simulink model "testemplanner_cs"  (R2020a)
settings: Solver=ode5  StartTime=0.0  StopTime=24  FixedStep=1/1000  RelTol=1e-3
PreLoadFcn:
  | mbxruntime.callbacks.PreLoadFcn(bdroot);
PostLoadFcn:
  | mbxruntime.callbacks.PostLoadFcn(bdroot);
InitFcn:
  | mbxruntime.callbacks.InitFcn(bdroot);
StartFcn:
  | mbxruntime.callbacks.StartFcn(bdroot);
StopFcn:
  | mbxruntime.callbacks.StopFcn(bdroot);
model workspace (MAT data in the model file):
  mbox_table : object (value not decoded)
  model_closed = 0
  sim_status = 0
values from neighbouring files (symbols this model uses):
  c_factor = 43.75    [emplanner_init.m]
  cf = -175016    [emplanner_init.m]
  cr = -130634    [emplanner_init.m]
  global_path_x = [0.057304 1.05668625507 2.05480936558 3.05165624935 4.04722112279 5.04150235808 6.03449985569 7.02621407764 8.01664569183 9.00579544113 9.99366409523 10.9802524329 ... (3001 elements, 3001x1)]    [global_path.mat]
  global_path_y = [8.29 8.29 8.29 8.29 8.29 8.29 8.29 8.29 8.29 8.29 8.29 8.29 ... (3001 elements, 3001x1)]    [global_path.mat]
  KD_PID_distance = 0.0    (= 0)    [emplanner_init.m]
  KD_PID_speed = 0    [emplanner_init.m]
  KI_PID_distance = 0.0    (= 0)    [emplanner_init.m]
  KI_PID_speed = 0    [emplanner_init.m]
  KP_PID_distance = 0.5    [emplanner_init.m]
  KP_PID_speed = 1.8    [emplanner_init.m]
  la = 1.265    [emplanner_init.m]
  lb = 2.947-1.265    (= 1.682)    [emplanner_init.m]
  LQR_K1 = k(:,1)'    [emplanner_init.m]
  LQR_K2 = k(:,2)'    [emplanner_init.m]
  LQR_K3 = k(:,3)'    [emplanner_init.m]
  LQR_K4 = k(:,4)'    [emplanner_init.m]
  m = 2020    [emplanner_init.m]
  rack_displacement = [-39.14 , -37.2 , -35.29 , -33.43 , -31.6 , -29.81 , -28.06 , -26.34 , -24.66 ,      -23.01 , -21.38 , -19.79 , -18.23 , -16.69 , -15.18 , -13.7 , -12.23 , -10.8 , -9.38 , -7.98 ,     -6.61 , -5.25 , -3.91 , -2.59 , -1.29 , 0 , 1.27 , 2.54 , 3.78 , 5.02 , 6.24 , 7.46 , 8.66 ,      9.86 , 11.05 , 12.24 , 13.41 , 14.59 , 15.76 , 16.92 , 18.09 , 19.25 , 20.42 , 21.59 , 22.76 ,      23.93 , 25.11 , 26 ...(+26 chars)    [emplanner_init.m]
  right_wheel_ground = [-70 ,-67.2 , -64.4 , -61.6 , -58.8 , -56 , -53.2 , -50.4 , -47.6 , -44.8 , -42 ,      -39.2 , -36.4 , -33.6 , -30.8 , -28 , -25.2 , -22.4 , -19.6 , -16.8 , -14 , -11.2 , -8.4 , -5.6 ,      -2.8 , 0 , 2.8 , 5.6 , 8.4 , 11.2 , 14 , 16.8 , 19.6 , 22.4 , 25.2 , 28 , 30.8 , 33.6 , 36.4 ,      39.2 , 42 , 44.8 , 47.6 , 50.4 , 53.2 , 56 , 58.8 , 61.6 , 64.4 , 67.2 , 70 ]    [emplanner_init.m]
  vx_break_point = zeros(1,5000)    [emplanner_init.m]
undefined symbols (not defined in the file or in its folder): aubr, DiscIntNeverNeededParam, tablebr, vubr
libraries: PreScanSimulinkLibrary x9, Solver_SF x1, simulink_extras x1
(part 5 of 9)

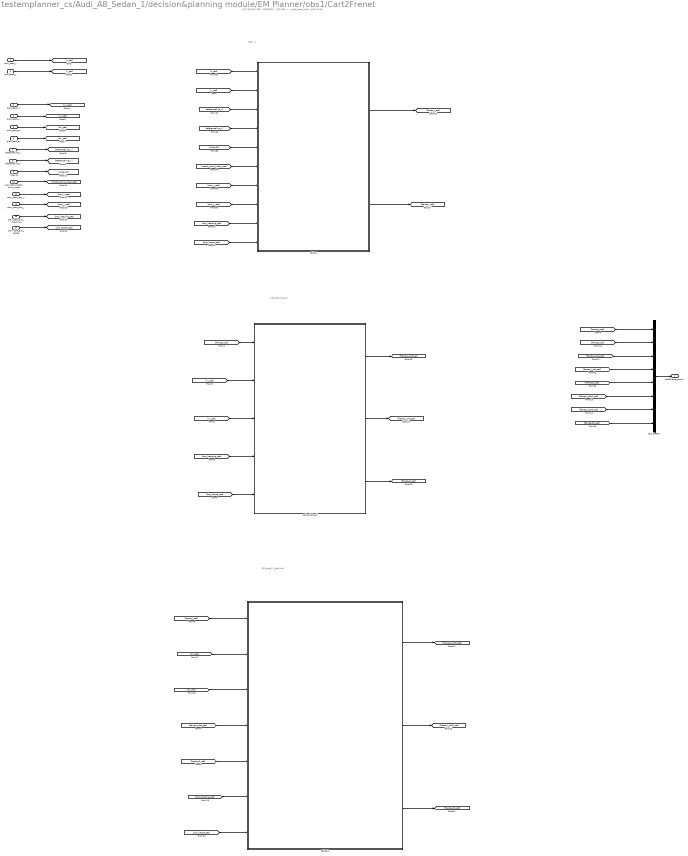
== system testemplanner_cs/Audi_A8_Sedan_1/decision&planning module/EM Planner/obs1/Cart2Frenet ==
  note: 计算s_dot_2,l_dot2,ddl
  note: 计算s_dot,l_dot,dl
  note: 计算S，L
  note: 分成三部分进行计算，方便后续拆分，分别计算S，L，s_dot,l_dot,s_dot2,l_dot2,dl和ddl
  plan_start_x : Inport
  plan_start_y : Inport  Port=2
  plan_start_vx : Inport  Port=3
  plan_start_vy : Inport  Port=4
  plan_start_ax : Inport  Port=5
  plan_start_ay : Inport  Port=6
  referenceline_x : Inport  Port=7
  referenceline_y : Inport  Port=8
  index2s : Inport  Port=9
  plan_start_match_point_index : Inport  Port=10
  plan_start_proj_x : Inport  Port=11
  plan_start_proj_y : Inport  Port=12
  plan_start_proj_heading : Inport  Port=13
  plan_start_proj_kappa : Inport  Port=14
  Bus Creator : BusCreator  Inputs=8
  CalcSL : MATLAB Function  TreatAsAtomicUnit=on
  CalcSL2 : MATLAB Function  TreatAsAtomicUnit=on
  Calcs_l_dot_dl : MATLAB Function  TreatAsAtomicUnit=on
  Cart2Frenet_result : Outport
  wires:
  Bus Creator/1 -> Cart2Frenet_result/1
  [frenet_ddl_set] -> Bus Creator/8
  [frenet_l_dot2_set] -> Bus Creator/7
  [frenet_s_dot2_set] -> Bus Creator/6
  [frenet_dl_set] -> Bus Creator/5
  [frenet_l_dot_set] -> Bus Creator/4
  [frenet_s_dot_set] -> Bus Creator/3
  [frenet_l_set] -> Bus Creator/2
  [frenet_s_set] -> Bus Creator/1
  CalcSL2/1(s_dot2_set) -> [frenet_s_dot2_set]
  CalcSL2/2(l_dot2_set) -> [frenet_l_dot2_set]
  CalcSL2/3(ddl_set) -> [frenet_ddl_set]
  [frenet_s_dot_set] -> CalcSL2/4(s_dot_set)
  [frenet_l_set] -> CalcSL2/1(frenet_l_set)
  [frenet_dl_set] -> CalcSL2/5(dl_set)
  [ay_set] -> CalcSL2/3(ay_set)
  [ax_set] -> CalcSL2/2(ax_set)
  Calcs_l_dot_dl/3(dl_set) -> [frenet_dl_set]
  Calcs_l_dot_dl/2(l_dot_set) -> [frenet_l_dot_set]
  Calcs_l_dot_dl/1(s_dot_set) -> [frenet_s_dot_set]
  [vy_set] -> Calcs_l_dot_dl/3(vy_set)
  [frenet_l_set] -> Calcs_l_dot_dl/1(frenet_l_set)
  CalcSL/2(frenet_l_set) -> [frenet_l_set]
  [proj_kappa_set] -> CalcSL2/7(plan_start_proj_kappa)
  [proj_heading_set] -> CalcSL2/6(plan_start_proj_heading)
  [vx_set] -> Calcs_l_dot_dl/2(vx_set)
  [proj_heading_set] -> Calcs_l_dot_dl/4(plan_start_proj_heading)
  [proj_kappa_set] -> Calcs_l_dot_dl/5(plan_start_proj_kappa)
  [proj_kappa_set] -> CalcSL/10(plan_start_proj_kappa)
  [proj_heading_set] -> CalcSL/9(plan_start_proj_heading)
  [proj_y_set] -> CalcSL/8(plan_start_proj_y)
  [proj_x_set] -> CalcSL/7(plan_start_proj_x)
  [match_point_index_set] -> CalcSL/6(plan_start_match_point_index)
  [index2s] -> CalcSL/5(index2s)
  [referenceline_y] -> CalcSL/4(referenceline_y)
  [referenceline_x] -> CalcSL/3(referenceline_x)
  [y_set] -> CalcSL/2(y_set)
  [x_set] -> CalcSL/1(x_set)
  plan_start_proj_kappa/1 -> [proj_kappa_set]
  plan_start_proj_heading/1 -> [proj_heading_set]
  plan_start_proj_y/1 -> [proj_y_set]
  plan_start_proj_x/1 -> [proj_x_set]
  plan_start_match_point_index/1 -> [match_point_index_set]
  index2s/1 -> [index2s]
  referenceline_y/1 -> [referenceline_y]
  referenceline_x/1 -> [referenceline_x]
  plan_start_ay/1 -> [ay_set]
  plan_start_ax/1 -> [ax_set]
  plan_start_vy/1 -> [vy_set]
  plan_start_vx/1 -> [vx_set]
  plan_start_y/1 -> [y_set]
  plan_start_x/1 -> [x_set]
  CalcSL/1(frenet_s_set) -> [frenet_s_set]

== system testemplanner_cs/Audi_A8_Sedan_1/decision&planning module/EM_planner1/obs/Cart2Frenet ==
  note: 计算s_dot_2,l_dot2,ddl
  note: 计算s_dot,l_dot,dl
  note: 计算S，L
  note: 分成三部分进行计算，方便后续拆分，分别计算S，L，s_dot,l_dot,s_dot2,l_dot2,dl和ddl
  plan_start_x : Inport
  plan_start_y : Inport  Port=2
  plan_start_vx : Inport  Port=3
  plan_start_vy : Inport  Port=4
  plan_start_ax : Inport  Port=5
  plan_start_ay : Inport  Port=6
  referenceline_x : Inport  Port=7
  referenceline_y : Inport  Port=8
  index2s : Inport  Port=9
  plan_start_match_point_index : Inport  Port=10
  plan_start_proj_x : Inport  Port=11
  plan_start_proj_y : Inport  Port=12
  plan_start_proj_heading : Inport  Port=13
  plan_start_proj_kappa : Inport  Port=14
  Bus Creator : BusCreator  Inputs=8
  CalcSL : MATLAB Function  TreatAsAtomicUnit=on
  CalcSL2 : MATLAB Function  TreatAsAtomicUnit=on
  Calcs_l_dot_dl : MATLAB Function  TreatAsAtomicUnit=on
  Cart2Frenet_result : Outport
  wires:
  Bus Creator/1 -> Cart2Frenet_result/1
  [frenet_ddl_set] -> Bus Creator/8
  [frenet_l_dot2_set] -> Bus Creator/7
  [frenet_s_dot2_set] -> Bus Creator/6
  [frenet_dl_set] -> Bus Creator/5
  [frenet_l_dot_set] -> Bus Creator/4
  [frenet_s_dot_set] -> Bus Creator/3
  [frenet_l_set] -> Bus Creator/2
  [frenet_s_set] -> Bus Creator/1
  CalcSL2/1(s_dot2_set) -> [frenet_s_dot2_set]
  CalcSL2/2(l_dot2_set) -> [frenet_l_dot2_set]
  CalcSL2/3(ddl_set) -> [frenet_ddl_set]
  [frenet_s_dot_set] -> CalcSL2/4(s_dot_set)
  [frenet_l_set] -> CalcSL2/1(frenet_l_set)
  [frenet_dl_set] -> CalcSL2/5(dl_set)
  [ay_set] -> CalcSL2/3(ay_set)
  [ax_set] -> CalcSL2/2(ax_set)
  Calcs_l_dot_dl/3(dl_set) -> [frenet_dl_set]
  Calcs_l_dot_dl/2(l_dot_set) -> [frenet_l_dot_set]
  Calcs_l_dot_dl/1(s_dot_set) -> [frenet_s_dot_set]
  [vy_set] -> Calcs_l_dot_dl/3(vy_set)
  [frenet_l_set] -> Calcs_l_dot_dl/1(frenet_l_set)
  CalcSL/2(frenet_l_set) -> [frenet_l_set]
  [proj_kappa_set] -> CalcSL2/7(plan_start_proj_kappa)
  [proj_heading_set] -> CalcSL2/6(plan_start_proj_heading)
  [vx_set] -> Calcs_l_dot_dl/2(vx_set)
  [proj_heading_set] -> Calcs_l_dot_dl/4(plan_start_proj_heading)
  [proj_kappa_set] -> Calcs_l_dot_dl/5(plan_start_proj_kappa)
  [proj_kappa_set] -> CalcSL/10(plan_start_proj_kappa)
  [proj_heading_set] -> CalcSL/9(plan_start_proj_heading)
  [proj_y_set] -> CalcSL/8(plan_start_proj_y)
  [proj_x_set] -> CalcSL/7(plan_start_proj_x)
  [match_point_index_set] -> CalcSL/6(plan_start_match_point_index)
  [index2s] -> CalcSL/5(index2s)
  [referenceline_y] -> CalcSL/4(referenceline_y)
  [referenceline_x] -> CalcSL/3(referenceline_x)
  [y_set] -> CalcSL/2(y_set)
  [x_set] -> CalcSL/1(x_set)
  plan_start_proj_kappa/1 -> [proj_kappa_set]
  plan_start_proj_heading/1 -> [proj_heading_set]
  plan_start_proj_y/1 -> [proj_y_set]
  plan_start_proj_x/1 -> [proj_x_set]
  plan_start_match_point_index/1 -> [match_point_index_set]
  index2s/1 -> [index2s]
  referenceline_y/1 -> [referenceline_y]
  referenceline_x/1 -> [referenceline_x]
  plan_start_ay/1 -> [ay_set]
  plan_start_ax/1 -> [ax_set]
  plan_start_vy/1 -> [vy_set]
  plan_start_vx/1 -> [vx_set]
  plan_start_y/1 -> [y_set]
  plan_start_x/1 -> [x_set]
  CalcSL/1(frenet_s_set) -> [frenet_s_set]

== system testemplanner_cs/Audi_A8_Sedan_1/Trajectories/Traj2State1/Traj2State2/Traj2MuxState_Ext/demux ==
  traj : Inport
  Demux : Demux  Outputs=18
  x : Outport
  y : Outport  Port=2
  z : Outport  Port=3
  velx : Outport  Port=4
  vely : Outport  Port=5
  velz : Outport  Port=6
  R : Outport  Port=7
  P : Outport  Port=8
  Y : Outport  Port=9
  velR : Outport  Port=10
  velP : Outport  Port=11
  velY : Outport  Port=12
  accx : Outport  Port=13
  accy : Outport  Port=14
  accz : Outport  Port=15
  accR : Outport  Port=16
  accP : Outport  Port=17
  accY : Outport  Port=18
  wires:
  Demux/18 -> accY/1
  Demux/17 -> accP/1
  Demux/16 -> accR/1
  Demux/15 -> accz/1
  Demux/14 -> accy/1
  Demux/13 -> accx/1
  Demux/12 -> velY/1
  Demux/11 -> velP/1
  Demux/10 -> velR/1
  Demux/9 -> velz/1
  Demux/8 -> vely/1
  Demux/7 -> velx/1
  Demux/6 -> Y/1
  Demux/5 -> P/1
  traj/1 -> Demux/1
  Demux/4 -> R/1
  Demux/3 -> z/1
  Demux/2 -> y/1
  Demux/1 -> x/1

== matlab function testemplanner_cs/Audi_A8_Sedan_1/decision&planning module/EM_planner1/calc speed planning start condition ==
  data: plan_start_vx input; plan_start_s_dot output; plan_start_vy input; plan_start_ax input; plan_start_ay input; plan_start_heading input; plan_start_s_dot2 output
function [plan_start_s_dot,plan_start_s_dot2] = fcn(plan_start_vx,plan_start_vy,plan_start_ax,plan_start_ay,plan_start_heading)
% 该函数计算速度规划的初始条件
tor = [cos(plan_start_heading);sin(plan_start_heading)];
v_t = tor'*[plan_start_vx;plan_start_vy];
a_t = tor'*[plan_start_ax;plan_start_ay];
plan_start_s_dot = v_t;
plan_start_s_dot2 = a_t;

== matlab function testemplanner_cs/Audi_A8_Sedan_1/decision&planning module/EM Planner/Cartesian2Frenet1/MATLAB Function2 ==
  data: ax_set input; s_dot2_set output; ay_set input; proj_heading_set input; proj_kappa_set input; l_set input; s_dot_set input; dl_set input; l_dot2_set output; ddl_set output
function [s_dot2_set,l_dot2_set,ddl_set] = fcn(ax_set,ay_set,proj_heading_set,proj_kappa_set,l_set,s_dot_set,dl_set)
%由于不知道有多少个点需要做坐标转换，设一个最大值做缓冲
n = 128;
% 输出初始化
s_dot2_set = ones(n,1)*nan;
l_dot2_set = ones(n,1)*nan;
ddl_set = ones(n,1)*nan;

for i = 1:length(l_set)
    if isnan(l_set(i))
       break;
    end
    a_h = [ax_set(i);ay_set(i)];
    n_r = [-sin(proj_heading_set(i));cos(proj_heading_set(i))];
    t_r = [cos(proj_heading_set(i));sin(proj_heading_set(i))];
    %近似认为dkr/ds 为0 简化计算
    l_dot2_set(i) = a_h'*n_r - proj_kappa_set(i) * (1 - proj_kappa_set(i) * l_set(i)) * s_dot_set(i)^2;
    s_dot2_set(i) = (1/(1 - proj_kappa_set(i) * l_set(i)))* (a_h' * t_r + 2 * proj_kappa_set(i) * dl_set(i) * s_dot_set(i)^2);
    % 要考虑加速度为0的情况
    if (s_dot2_set(i) < 1e-6)
        ddl_set(i) = 0;
    else
        ddl_set(i) = (l_dot2_set(i) - dl_set(i)*s_dot2_set(i))/(s_dot_set(i)^2);
    end
end

== matlab function testemplanner_cs/Audi_A8_Sedan_1/decision&planning module/EM_planner1/general fast algorithm to find projection point info3 ==
  data: x_set input; match_point_index_set output; y_set input; path_x input; path_y input; proj_x_set output; proj_y_set output; proj_heading_set output; proj_kappa_set output; path_heading input; path_kappa input
function [match_point_index_set,proj_x_set,proj_y_set,proj_heading_set,proj_kappa_set] = fcn(x_set,y_set,path_x,path_y,path_heading,path_kappa)
%该函数是一个通用函数，找到x_set,y_set在path_x,path_y的匹配点的编号，以及投影点在直角坐标系下的(x,y,theta,kappa)
%最多可以处理128个点

match_point_index_set = ones(128,1)*nan;
proj_x_set = ones(128,1)*nan;
proj_y_set = ones(128,1)*nan;
proj_heading_set = ones(128,1)*nan;
proj_kappa_set = ones(128,1)*nan;

persistent is_first_run;
persistent init_search_index_set;
persistent pre_frenet_path_x;
persistent pre_frenet_path_y;
persistent pre_frenet_path_heading;
persistent pre_frenet_path_kappa;
if isempty(is_first_run)
    is_first_run = 0; 
    init_search_index_set = ones(128,1)*nan;
    start_index = 1;
    pre_frenet_path_x = path_x;
    pre_frenet_path_y = path_y;
    pre_frenet_path_heading = path_heading;
    pre_frenet_path_kappa = path_kappa;
    for i = 1:length(x_set)
        if isnan(x_set(i))
            break;
        else
            increase_count = 0;
            min_distance = 1e10;
            for j = start_index:length(path_x)
                distance = (x_set(i)-path_x(j))^2 + (y_set(i)-path_y(j))^2;
                if (min_distance > distance)
                    min_distance = distance;
                    match_point_index_set(i)=j;
                    increase_count = 0;
                else
                    increase_count = increase_count + 1;
                end
                if increase_count > 50
                    break;
                end
            end
            match_point_index = match_point_index_set(i);
            vector_match_point = [path_x(match_point_index);path_y(match_point_index)];
            vector_match_point_direction = [cos(path_heading(match_point_index));sin(path_heading(match_point_index))];
            vector_host_point = [x_set(i);y_set(i)];
            vector_d = vector_host_point - vector_match_point;
            vector_err = (vector_d'* vector_match_point_direction) * vector_match_point_direction;
            vector_proj = vector_err + vector_match_point;
            proj_x_set(i) = vector_proj(1);
            proj_y_set(i) = vector_proj(2);
            proj_heading_set(i) = path_heading(match_point_index) + path_kappa(match_point_index) * (vector_d'* vector_match_point_direction);
            proj_kappa_set(i) = path_kappa(match_point_index);            
        end
    end 
    init_search_index_set=match_point_index_set;
else
    min_distance = inf;
    for i = 1:length(x_set)
        increase_count = 0;
        count_limit=5;
        if isnan(init_search_index_set(i))
            start_index = 1;
            count_limit=50;
       
        
        else
            
            start_index = init_search_index_set(i);
          
         end  
            
            vector_m_init = [pre_frenet_path_x(start_index);pre_frenet_path_y(start_index)];
            vector_direction_init = [cos(pre_frenet_path_heading(start_index));sin(pre_frenet_path_heading(start_index))];
            ds = vector_m_init'*vector_direction_init;
            if ds > 0.001            
                for j = start_index:length(pre_frenet_path_x )
                    distance = (x_set(i)-pre_frenet_path_x (j))^2 + (y_set(i)-pre_frenet_path_y(j))^2;
                    if (min_distance > distance)
                        min_distance = distance;
                        init_search_index_set(i)=j;
                        increase_count = 0;
                    else
                        increase_count = increase_count + 1;
                    end
                    if increase_count > count_limit
                        break;
                    end
                end
            elseif ds < -0.001
                for j = start_index:-1:1
                    distance = (x_set(i)-pre_frenet_path_x (j))^2 + (y_set(i)-pre_frenet_path_y(j))^2;
                    if (min_distance > distance)
                        min_distance = distance;
                        init_search_index_set(i)=j;
                        increase_count = 0;
                    else
                        increase_count = increase_count + 1;
                    end
                    if increase_count >  count_limit
                        break;
                    end
                end
              match_point_index_set(i)=start_index;  
            end
            
           match_point_index= match_point_index_set(i);
            vector_match_point = [pre_frenet_path_x(match_point_index);pre_frenet_path_y(match_point_index)];
            vector_match_point_direction = [cos(pre_frenet_path_heading(match_point_index));sin(pre_frenet_path_heading(match_point_index))];
            vector_host_point = [x_set(i);y_set(i)];
            vector_d = vector_host_point - vector_match_point;
            vector_err = (vector_d'* vector_match_point_direction) * vector_match_point_direction;
            vector_proj = vector_err + vector_match_point;
            proj_x_set(i) = vector_proj(1);
            proj_y_set(i) = vector_proj(2);
            proj_heading_set(i) = pre_frenet_path_heading(match_point_index) + pre_frenet_path_kappa(match_point_index) * (vector_d'* vector_match_point_direction);
            proj_kappa_set(i) = pre_frenet_path_kappa(match_point_index);            
        end
    end    
    init_search_index_set = match_point_index_set;
    pre_frenet_path_x = path_x;
    pre_frenet_path_y = path_y;
    pre_frenet_path_heading = path_heading;
    pre_frenet_path_kappa = path_kappa;
end

== matlab function testemplanner_cs/Audi_A8_Sedan_1/decision&planning module/EM_planner1/increase st point count ==
  data: s_init input; s output; s_dot_init input; s_dot2_init input; relative_time_init input; s_dot output; s_dot2 output; relative_time output
function [s,s_dot,s_dot2,relative_time] = fcn(s_init,s_dot_init,s_dot2_init,relative_time_init)
%该函数将增密s s_dot s_dot2
% 为什么需要增密，因为控制的执行频率是规划的10倍，轨迹点如果不够密，必然会导致规划效果不好
% 但是若在速度二次规划中点取的太多，会导致二次规划的矩阵规模太大计算太慢
% 所以方法是在二次规划中选取少量的点优化完毕后，在用此函数增密
T = relative_time_init(end);
n = 401;
dt = T/(n-1);
s = zeros(n,1);
s_dot = zeros(n,1);
s_dot2 = zeros(n,1);
relative_time = zeros(n,1);
for i = 1:n
    current_t = (i-1)*dt;
    for j = 1:length(relative_time_init)-1
        if relative_time_init(j) <= current_t && relative_time_init(j+1) > current_t
            break;
        end
    end
    x = current_t - relative_time_init(j);
    s(i) = s_init(j) + s_dot_init(j)*x + (1/3)*s_dot2_init(j)*x^2 + (1/6)*s_dot2_init(j+1)*x^2; 
    s_dot(i) = s_dot_init(j) + 0.5*s_dot2_init(j)*x + 0.5*s_dot2_init(j+1)*x;
    s_dot2(i) = s_dot2_init(j) + (s_dot2_init(j+1) - s_dot2_init(j))*x/(relative_time_init(j+1) - relative_time_init(j));
    relative_time(i) = current_t;
end

== matlab function testemplanner_cs/Audi_A8_Sedan_1/decision&planning module/EM_planner1/obs/Cart2Frenet/CalcSL ==
  data: x_set input; y_set input; referenceline_x input; referenceline_y input; index2s input; plan_start_match_point_index input; plan_start_proj_x input; plan_start_proj_y input; plan_start_proj_heading input; plan_start_proj_kappa input; frenet_s_set output; frenet_l_set output
function [frenet_s_set,frenet_l_set] =fcn(x_set,y_set,referenceline_x,referenceline_y,index2s,plan_start_match_point_index,plan_start_proj_x,plan_start_proj_y,plan_start_proj_heading,plan_start_proj_kappa)
%作用：这是一个通用函数，计算输入的笛卡尔坐标点x,y在自然坐标（frenet）坐标系中的s和l
%输入:要计算的点集的x,y坐标，航向，曲率。他的投影点的x,y坐标，index2s数据，以及参考线数据
%输出：自然坐标系下的s和l
%首先对s和l做一个缓冲
frenet_s_set=ones(128,1)*nan;
frenet_l_set=ones(128,1)*nan;
%开始计算
for i=1:length(x_set)
if isnan(x_set(i))  %遇到空的跳出
    break;
end
%调用相关函数进行s的计算
frenet_s_set(i)=CalcSfromIndex(referenceline_x,referenceline_y,plan_start_proj_x(i),plan_start_proj_y(i),plan_start_match_point_index(i),index2s);

%进行l的计算
%先求自然坐标系的切向量和法向量
%切向量,没用到
%tor=[cos(plan_start_proj_heading(i));sin(plan_start_proj_heading(i))];
%法向量
nor=[-sin(plan_start_proj_heading(i));cos(plan_start_proj_heading(i))];
frenet_l_set(i)=[x_set(i)-plan_start_proj_x(i);y_set(i)-plan_start_proj_y(i)]'*nor;
end

end
function s=CalcSfromIndex(ref_path_x,ref_path_y,match_point_x,match_point_y,match_point_index,index2s)   %使用一个函数来计算index所对应的S值
%%首先判断原点是在匹配点前还是匹配点后，通过向量的内积来进行判断
s_temp =  index2s(match_point_index);
vector1=[match_point_x-ref_path_x(match_point_index);match_point_y-ref_path_y(match_point_index)];
%考虑匹配点在路径终点的情况，不在终点就是匹配点和下一个点作为方向向量，如果是终点则使用匹配点和上一个点作为方向向量
if match_point_index<length(ref_path_x)
    vector2=[ref_path_x(match_point_index+1)-ref_path_x(match_point_index);ref_path_y(match_point_index+1)-ref_path_y(match_point_index)];
else
     vector2=[ref_path_x(match_point_index)-ref_path_x(match_point_index-1);ref_path_y(match_point_index)-ref_path_y(match_point_index-1)];
end
result=vector1'*vector2;    
if result >0 %原点在匹配点后，加上这个距离
    s=s_temp+sqrt(vector1'*vector1);
else        %原点在匹配点前，减去这个距离
    s=s_temp-sqrt(vector1'*vector1);
end
end

== matlab function testemplanner_cs/Audi_A8_Sedan_1/decision&planning module/EM_planner1/obs/Cart2Frenet/CalcSL2 ==
  data: frenet_l_set input; ax_set input; ay_set input; s_dot_set input; dl_set input; plan_start_proj_heading input; plan_start_proj_kappa input; s_dot2_set output; l_dot2_set output; ddl_set output
function [ s_dot2_set, l_dot2_set,ddl_set]=fcn(frenet_l_set,ax_set,ay_set,s_dot_set,dl_set,plan_start_proj_heading,plan_start_proj_kappa)
%作用：通过之前计算得到的l，s_dot、dl值以及已知的ax，ay值，计算s_dot2,l_dot2,以及ddl
 %首先做一个缓冲
 n=128;
 s_dot2_set=ones(n,1)*nan;
 l_dot2_set=ones(n,1)*nan;
 ddl_set=ones(n,1)*nan;

 for i=1:length(frenet_l_set)
     if isnan(frenet_l_set(i))
         break;
     end
    %先求自然坐标系的切向量和法向量
%切向量
tor=[cos(plan_start_proj_heading(i));sin(plan_start_proj_heading(i))];
%法向量
nor=[-sin(plan_start_proj_heading(i));cos(plan_start_proj_heading(i))];

ah=[ax_set(i);ay_set(i)];
l_dot2_set(i)=ah'*nor- plan_start_proj_kappa(i) * (1 - plan_start_proj_kappa(i) * frenet_l_set(i)) * s_dot_set(i)^2;
s_dot2_set(i)=(1/(1 - plan_start_proj_kappa(i) * frenet_l_set(i)))* (ah' * tor + 2 * plan_start_proj_kappa(i) * dl_set(i) * s_dot_set(i)^2);

if abs(s_dot2_set(i))<1e-6
    ddl_set(i)=0;
else
    ddl_set(i)=(l_dot2_set(i) - dl_set(i)*s_dot2_set(i))/(s_dot_set(i)^2);
 end
end

== matlab function testemplanner_cs/Audi_A8_Sedan_1/decision&planning module/EM_planner1/obs/Cart2Frenet/Calcs_l_dot_dl ==
  data: frenet_l_set input; vx_set input; vy_set input; plan_start_proj_heading input; plan_start_proj_kappa input; s_dot_set output; l_dot_set output; dl_set output
function [ s_dot_set, l_dot_set,dl_set]=fcn(frenet_l_set,vx_set,vy_set,plan_start_proj_heading,plan_start_proj_kappa)
%作用：通过之前计算得到的s和l值以及计算的速度值，计算s_dot,l_dot,以及dl
 %首先做一个缓冲
 n=128;
 s_dot_set=ones(n,1)*nan;
 l_dot_set=ones(n,1)*nan;
 dl_set=ones(n,1)*nan;

 for i=1:length(frenet_l_set)
     if isnan(frenet_l_set(i))
         break;
     end
    %先求自然坐标系的切向量和法向量
%切向量
tor=[cos(plan_start_proj_heading(i));sin(plan_start_proj_heading(i))];
%法向量
nor=[-sin(plan_start_proj_heading(i));cos(plan_start_proj_heading(i))];

vh=[vx_set(i);vy_set(i)];
l_dot_set(i)=vh'*nor;
s_dot_set(i)=vh'*tor/(1-plan_start_proj_kappa(i)*frenet_l_set(i));

if abs(s_dot_set(i))<1e-6
    dl_set(i)=0;
else
    dl_set(i)=l_dot_set(i)/s_dot_set(i);
 end
end

== matlab function testemplanner_cs/Audi_A8_Sedan_1/decision&planning module/EM_planner1/obs/MATLAB Function2 ==
  data: x_set input; match_point_index_set output; y_set input; frenet_path_x input; frenet_path_y input; frenet_path_heading input; frenet_path_kappa input; proj_x_set output; proj_y_set output; proj_heading_set output; proj_kappa_set output
function [match_point_index_set,proj_x_set, proj_y_set,proj_heading_set,proj_kappa_set] = ...
    fcn(x_set,y_set,frenet_path_x,frenet_path_y,frenet_path_heading,frenet_path_kappa)
%该函数将批量计算x_set，y_set中的xy，在frenet_path下的投影的信息
%输入 x_set,y_set，待投影的点的集合
%x_set,y_set,frenet_path_x,frenet_path_y,frenet_path_heading,frenet_path_kappa
%曲线在直角坐标系下的x，y，heading，kappa
%输出：match_point_index_set 匹配点在frenet_path下的编号的集合(即从全局路径第一个点开始数，第几个点是匹配点)
%     proj_x y heading kappa 投影的x,y,heading,kappa的集合

% 由于事先不知道x_set中到底有多少个点需要投影，因此事先声明一个最大的数量的点作为缓冲
n = 128;
% 并且由于不知道投影点的个数，所以也不知道输出的个数，因此输出也要做缓冲，用nan表示不存在的点
% 输出最多输出128个
% 输出初始化
match_point_index_set = ones(n,1) * nan;
proj_x_set = ones(n,1) * nan;
proj_y_set = ones(n,1) * nan;
proj_heading_set = ones(n,1) * nan;
proj_kappa_set = ones(n,1) * nan;

%找匹配点，需要利用上一个周期的结果作为下一个周期遍历的起点，因此需要声明两个全局变量
persistent is_first_run;
persistent pre_match_point_index_set;
persistent pre_frenet_path_x;
persistent pre_frenet_path_y;
persistent pre_frenet_path_heading;
persistent pre_frenet_path_kappa;
%算法主函数入口

if isempty(is_first_run)
    %该if分支表示函数首次运行
    is_first_run = 0;
    pre_frenet_path_x = frenet_path_x;
    pre_frenet_path_y = frenet_path_y;
    pre_frenet_path_heading = frenet_path_heading;
    pre_frenet_path_kappa = frenet_path_kappa;
    %要记录首次运行计算的匹配点的结果供下个周期运行，先初始化
    pre_match_point_index_set = ones(n,1) * nan;
    %对x_set,y_set的点做遍历，找到他们的匹配点
    for i = 1 : length(x_set)
        if isnan(x_set(i))
            break;
        end
        %首次运行时，没有任何提示，只能从frenet path的第一个点开始找
        start_search_index = 1;
        % 声明increase_count，用于表示在遍历时distance连续增加的个数
        increase_count = 0;
        % 开始遍历
        min_distance = inf;
        for j = start_search_index : length(frenet_path_x)
            distance = (x_set(i) - frenet_path_x(j))^2 + (y_set(i) - frenet_path_y(j))^2;
            if distance < min_distance
                min_distance = distance;
                match_point_index_set(i) = j;
                increase_count = 0;
            else
                increase_count = increase_count + 1;
            end
            %如果distance连续增加50次就不要再遍历了，节省时间
            if increase_count > 50
                break;
            end
        end
        
        %如何通过匹配点计算投影点，请参见《自动驾驶控制算法第七讲》
        %或《自动驾驶决策规划算法》第一章第三节
        
        %取出匹配点的编号
        match_point_index = match_point_index_set(i);
        %取出匹配点的信息
        match_point_x = frenet_path_x(match_point_index);
        match_point_y = frenet_path_y(match_point_index);
        match_point_heading = frenet_path_heading(match_point_index);
        match_point_kappa = frenet_path_kappa(match_point_index);
        %计算匹配点的方向向量与法向量
        vector_match_point = [match_point_x;match_point_y];
        vector_match_point_direction = [cos(match_point_heading);sin(match_point_heading)];
        %声明待投影点的位矢
        vector_r = [x_set(i);y_set(i)];
        
       %通过匹配点计算投影点
       vector_d = vector_r - vector_match_point;
       ds = vector_d' * vector_match_point_direction;
       vector_proj_point = vector_match_point + ds * vector_match_point_direction;
       proj_heading = match_point_heading + match_point_kappa * ds;
       proj_kappa = match_point_kappa;
       %计算结果输出
       proj_x_set(i) = vector_proj_point(1);
       proj_y_set(i) = vector_proj_point(2);
       proj_heading_set(i) = proj_heading;
       proj_kappa_set(i) = proj_kappa;
    end
    %匹配点的计算结果保存，供下一个周期使用
    pre_match_point_index_set = match_point_index_set;
else
    %此if分支表示不是首次运行
    
    %对每个x_set上的点做处理
    for i = 1 : length(x_set)
        %不是首次运行，对于点x_set(i),y_set(i)来说,start_search_index =
        %pre_match_point_index_set(i)
        start_search_index = pre_match_point_index_set(i);%上个周期匹配点的编号作为本周期搜索的起点
        % 声明increase_count，用于表示在遍历时distance连续增加的个数
        %%%%%%%%%
        %对于障碍物检测而言，当感知第一次检测到障碍物时，算法并不是首次运行，此时 
        %pre_match_point_index_set的值是nan，如果还用上一时刻的结果作为本周期搜索的起点
        %必然会出问题，所以要修改
        % 声明increase_count_limit
        increase_count_limit = 5;
        if isnan(start_search_index)
            %没有上个周期的结果，那就不能只检查5次了
            increase_count_limit = 50;
            %搜索起点也要设为1
            start_search_index = 1;
        end
        increase_count = 0;
        % 开始遍历
        %这里多一个步骤，判断遍历的方向
        %计算上个周期匹配点的位矢
        vector_pre_match_point = [pre_frenet_path_x(start_search_index);pre_frenet_path_y(start_search_index)];
        vector_pre_match_point_direction = ...
            [cos(pre_frenet_path_heading(start_search_index));sin(pre_frenet_path_heading(start_search_index))];
        %判断遍历的方向
        flag = ([x_set(i);y_set(i)] - vector_pre_match_point)' * vector_pre_match_point_direction;
        min_distance = inf;
        if flag > 0.001
            for j = start_search_index : length(frenet_path_x)
                distance = (x_set(i) - frenet_path_x(j))^2 + (y_set(i) - frenet_path_y(j))^2;
                if distance < min_distance
                    min_distance = distance;
                    match_point_index_set(i) = j;
                    increase_count = 0;
                else
                    increase_count = increase_count + 1;
                end
                %如果distance连续增加increase_count_limit次就不要再遍历了，节省时间
                if increase_count > increase_count_limit
                    break;
                end
            end
        elseif flag < - 0.001
            for j = start_search_index : -1 : 1
                distance = (x_set(i) - frenet_path_x(j))^2 + (y_set(i) - frenet_path_y(j))^2;
                if distance < min_distance
                    min_distance = distance;
                    match_point_index_set(i) = j;
                    increase_count = 0;
                else
                    increase_count = increase_count + 1;
                end
                %如果distance连续增加increase_count_limit次就不要再遍历了，节省时间
                if increase_count > increase_count_limit
                    break;
                end
            end
        else
            match_point_index_set(i) = start_search_index;
        end
        
        %如何通过匹配点计算投影点，请参见《自动驾驶控制算法第七讲》
        %或《自动驾驶决策规划算法》第一章第三节
        
        %取出匹配点的编号
        match_point_index = match_point_index_set(i);
        %取出匹配点的信息
        match_point_x = frenet_path_x(match_point_index);
        match_point_y = frenet_path_y(match_point_index);
        match_point_heading = frenet_path_heading(match_point_index);
        match_point_kappa = frenet_path_kappa(match_point_index);
        %计算匹配点的方向向量与法向量
        vector_match_point = [match_point_x;match_point_y];
        vector_match_point_direction = [cos(match_point_heading);sin(match_point_heading)];
        %声明待投影点的位矢
        vector_r = [x_set(i);y_set(i)];
        
       %通过匹配点计算投影点
       vector_d = vector_r - vector_match_point;
       ds = vector_d' * vector_match_point_direction;
       vector_proj_point = vector_match_point + ds * vector_match_point_direction;
       proj_heading = match_point_heading + match_point_kappa * ds;
       proj_kappa = match_point_kappa;
       %计算结果输出
       proj_x_set(i) = vector_proj_point(1);
       proj_y_set(i) = vector_proj_point(2);
       proj_heading_set(i) = proj_heading;
       proj_kappa_set(i) = proj_kappa;
  
    end
    %匹配点的计算结果保存，供下一个周期使用
    pre_match_point_index_set = match_point_index_set;
    pre_frenet_path_x = frenet_path_x;
    pre_frenet_path_y = frenet_path_y;
    pre_frenet_path_heading = frenet_path_heading;
    pre_frenet_path_kappa = frenet_path_kappa;
end

== matlab function testemplanner_cs/Audi_A8_Sedan_1/decision&planning module/EM_planner1/obs/obs_fliter ==
  data: host_x input; obs_x_set_gcs_afterfliter output; host_y input; host_heading_xy input; obs_x_set_gcs input; obs_y_set_gcs input; obs_velocity_set_gcs input; obs_heading_set_gcs input; obs_y_set_gcs_afterfliter output; obs_velocity_set_gcs_afterfliter output; obs_heading_set_gcs_afterfliter output
function [obs_x_set_gcs_afterfliter,obs_y_set_gcs_afterfliter,obs_velocity_set_gcs_afterfliter,obs_heading_set_gcs_afterfliter] = fcn(host_x,host_y,host_heading_xy,obs_x_set_gcs,obs_y_set_gcs,obs_velocity_set_gcs,obs_heading_set_gcs)
%%作用：进行障碍筛选，只有在车辆纵向距离为[-10,60],横向距离为[-10，10]的障碍物才被处理
%%输入：车辆的坐标和航向，障碍物的坐标、速度和航向
%%输出：经过筛选后的障碍物的坐标、速度和航向

%%首先做一个缓冲
n=32; %只使用32个障碍物
obs_x_set_gcs_afterfliter=ones(n,1)*nan;
obs_y_set_gcs_afterfliter=ones(n,1)*nan;
obs_velocity_set_gcs_afterfliter=ones(n,1)*nan;
obs_heading_set_gcs_afterfliter=ones(n,1)*nan;
count=1;
%%
for i=1:length(obs_x_set_gcs)
    if isnan(obs_x_set_gcs(i))
        break;
    end
      %先求车辆坐标系的切向量和法向量
%切向量
tor=[cos(host_heading_xy(i));sin(host_heading_xy(i))];
%法向量
nor=[-sin(host_heading_xy(i));cos(host_heading_xy(i))];

lon_distance = [obs_x_set_gcs(i)-host_x;obs_y_set_gcs(i)-host_y]'*tor;
lat_distance = [obs_x_set_gcs(i)-host_x;obs_y_set_gcs(i)-host_y]'*nor;

if lon_distance>=-10 && lon_distance<=60&&lat_distance>=-10 && lat_distance<=10
    obs_x_set_gcs_afterfliter(count)=obs_x_set_gcs(i);
    obs_y_set_gcs_afterfliter(count)=obs_y_set_gcs(i);
    obs_velocity_set_gcs_afterfliter(count)=obs_velocity_set_gcs(i);
    obs_heading_set_gcs_afterfliter(count)=obs_heading_set_gcs(i);
    count=count+1;
end
end

== matlab function testemplanner_cs/Audi_A8_Sedan_1/decision&planning module/EM_planner1/obs/obs_fliter_for_static ==
  data: obs_x_set_gcs_afterfliter input; obs_x_set_gcs_static output; obs_y_set_gcs_afterfliter input; obs_velocity_set_gcs_afterfliter input; obs_heading_set_gcs_afterfliter input; obs_y_set_gcs_static output; obs_x_set_gcs_dynamic output; obs_y_set_gcs_dynamic output; obs_velocity_set_gcs_dynamic output; obs_heading_set_gcs_dynamic output
function [obs_x_set_gcs_static,obs_y_set_gcs_static,obs_x_set_gcs_dynamic,obs_y_set_gcs_dynamic,obs_velocity_set_gcs_dynamic,obs_heading_set_gcs_dynamic] = fcn(obs_x_set_gcs_afterfliter,obs_y_set_gcs_afterfliter,obs_velocity_set_gcs_afterfliter,obs_heading_set_gcs_afterfliter)
%%作用：进行障碍筛选，只有在车辆纵向距离为[-10,60],横向距离为[-10，10]的障碍物才被处理
%%输入：车辆的坐标和航向，障碍物的坐标、速度和航向
%%输出：经过筛选后的障碍物的坐标、速度和航向

%%首先做一个缓冲
n=32; %只使用32个障碍物
obs_x_set_gcs_static=ones(n,1)*nan;
obs_y_set_gcs_static=ones(n,1)*nan;
obs_x_set_gcs_dynamic=ones(n,1)*nan;
obs_y_set_gcs_dynamic=ones(n,1)*nan;
obs_velocity_set_gcs_dynamic=ones(n,1)*nan;
obs_heading_set_gcs_dynamic=ones(n,1)*nan;
count_static=1;
count_dynamic=1;
%%
for i=1:length(obs_x_set_gcs_afterfliter)
   
if abs(obs_velocity_set_gcs_afterfliter)<0.1
    obs_x_set_gcs_static(count_static)=obs_x_set_gcs_afterfliter(i);
    obs_y_set_gcs_static(count_static)=obs_y_set_gcs_afterfliter(i);
    count_static=count_static+1;
else
    obs_x_set_gcs_dynamic(count_dynamic)=obs_x_set_gcs_afterfliter(i);
    obs_y_set_gcs_dynamic(count_dynamic)=obs_y_set_gcs_afterfliter(i);
    obs_velocity_set_gcs_dynamic(count_dynamic)=obs_velocity_set_gcs_afterfliter(i)*cos(obs_heading_set_gcs_afterfliter(i));
    obs_heading_set_gcs_dynamic(count_dynamic)=obs_velocity_set_gcs_afterfliter(i)*sin(obs_heading_set_gcs_afterfliter(i));
    count_dynamic=count_dynamic+1;
end
end

== matlab function testemplanner_cs/Audi_A8_Sedan_1/decision&planning module/EM_planner1/path and speed merge ==
  data: s input; trajectory_x output; s_dot input; s_dot2 input; relative_time input; current_time input; path_s input; trajectory_x_init input; trajectory_y_init input; trajectory_heading_init input; trajectory_kappa_init input; trajectory_y output; trajectory_heading output; trajectory_kappa output; trajectory_speed output; trajectory_accel output; trajectory_time output
function [trajectory_x,trajectory_y,trajectory_heading,trajectory_kappa,trajectory_speed,trajectory_accel,trajectory_time] = ...
    fcn(s,s_dot,s_dot2,relative_time,current_time,path_s,trajectory_x_init,trajectory_y_init,trajectory_heading_init,trajectory_kappa_init)
% 该函数将合并path和speed
% 由于path 是 60个点，speed 有 401个点，合并后，path和speed有401个点，因此需要做插值
n = 401;
trajectory_x = zeros(n,1);
trajectory_y = zeros(n,1);
trajectory_heading = zeros(n,1);
trajectory_kappa = zeros(n,1);
trajectory_speed = zeros(n,1);

trajectory_accel = zeros(n,1);
index = 1;
% 由于trajectory_x_init中不是所有的值都有效，(有nan) 所以要找到有效值的范围
while ~isnan(trajectory_x_init(index)) 
    index = index + 1;
end
index = index - 1;
trajectory_time = zeros(n,1);
for i = 1:n-1
    %interp1 线性插值
    % 若 x = [1,2] y = [3,4]
    %interp1(x,y,1.5) 会得到3.5
    %interp1 的缺点是 在端点或超过端点的，结果为nan
    % interp1(x,y,2) 不会等于4 而是会等于nan
    % interp1(x,y,6) 也会等于nan，所以在端点处要单独处理
    trajectory_x(i) = interp1(path_s(1:index),trajectory_x_init(1:index),s(i));
    trajectory_y(i) = interp1(path_s(1:index),trajectory_y_init(1:index),s(i));
    trajectory_heading(i) = interp1(path_s(1:index),trajectory_heading_init(1:index),s(i));
    trajectory_kappa(i) = interp1(path_s(1:index),trajectory_kappa_init(1:index),s(i));
    trajectory_time(i) = relative_time(i) + current_time;%速度规划会得到相对时间，转换成绝对时间
    trajectory_speed(i) = s_dot(i);
    trajectory_accel(i) = s_dot2(i);
end
% 端点单独处理
trajectory_x(end) = trajectory_x_init(end);
trajectory_y(end) = trajectory_y_init(end);
trajectory_heading(end) = trajectory_heading_init(end);
trajectory_kappa(end) = trajectory_kappa_init(end);
trajectory_time(end) = relative_time(end) + current_time;
trajectory_speed(end) = s_dot(end);
trajectory_accel(end) = s_dot2(end);

== matlab function testemplanner_cs/Audi_A8_Sedan_1/decision&planning module/EM Planner/DP node generate1 ==
  data: dp_path_s_init input; dp_path_s_final output; dp_path_l_init input; plan_start_s input; plan_start_l input; plan_start_dl input; plan_start_ddl input; dp_path_l_final output; dp_path_dl_final output; dp_path_ddl_final output
function [dp_path_s_final,dp_path_l_final,dp_path_dl_final,dp_path_ddl_final] = fcn(dp_path_s_init,dp_path_l_init,plan_start_s,plan_start_l,plan_start_dl,plan_start_ddl)
%%作用：对DP求得的路径进行路径点加密
%%输入：dp求得的点s，l参数，规划起点的s，l，dl，ddl参数
%%输出：加密后的路径点的s，l，dl，ddl参数
%每隔1m取一个点
ds=1;
%初始化输出数组
dp_path_s_final=ones(60,1)*nan;
dp_path_l_final=ones(60,1)*nan;
dp_path_dl_final=ones(60,1)*nan;
dp_path_ddl_final=ones(60,1)*nan;

%初始化过程变量
cur_node_s=0;
l_temp=[];
dl_temp=[];
ddl_temp=[];
%初始化路径起点
start_s=plan_start_s;
start_l=plan_start_l;
start_dl=plan_start_dl;
start_ddl=plan_start_ddl;
%遍历整个输入的s集合，进行节点加密
for i=1:length(dp_path_s_init)
    if dp_path_s_init==-1
        break;
    end
    end_s=dp_path_s_init(i);
    end_l=dp_path_l_init(i);
    end_dl=0;
    end_ddl=0;
    coffee=Calccoffee(start_s,start_l,start_dl,start_ddl,end_s,end_l,end_dl,end_ddl);
    for j=1:10000
        if(start_s+ds*(j-1))<end_s
            cur_node_s=start_s+ds*(j-1);
            l_cur=coffee(6)*(cur_node_s)^5+coffee(5)*(cur_node_s)^4+coffee(4)*(cur_node_s)^3+coffee(3)*(cur_node_s)^2+coffee(2)*(cur_node_s)+coffee(1);
            dl_cur=5*coffee(6)*(cur_node_s)^4+4*coffee(5)*(cur_node_s)^3+3*coffee(4)*(cur_node_s)^2+2*coffee(3)*(cur_node_s)+coffee(2);
            ddl_cur=20*coffee(6)*(cur_node_s)^3+12*coffee(5)*(cur_node_s)^2+6*coffee(4)*(cur_node_s)+2*coffee(3);
            l_temp=[l_temp,l_cur];
            dl_temp=[dl_temp,dl_cur];
            ddl_temp=[ddl_temp,ddl_cur];
            
        else
            break;
        end
    end
      start_s=end_s;
      start_l=end_l;
      start_dl=end_dl;
      start_ddl=end_ddl;
end

for k=1:length(l_temp)
    if k==61
        break;
    else
        dp_path_s_final(k)=plan_start_s+ds*(k-1);
        dp_path_l_final(k)=l_temp(k);
        dp_path_dl_final(k)=dl_temp(k);
        dp_path_ddl_final(k)=ddl_temp(k);
    end
end

end

function coffee=Calccoffee(start_s,start_l,start_dl,start_ddl,end_s,end_l,end_dl,end_ddl)
  %作用：计算五次多项式系数
  %输入：起点和终点的s,l,dl,ddl共6个值
  %输出：六个权重系数
    start_s2=start_s*start_s;
    start_s3=start_s2*start_s;
    start_s4=start_s3*start_s;
    start_s5=start_s4*start_s;
    end_s2=end_s*end_s;
    end_s3=end_s2*end_s;
    end_s4=end_s3*end_s;
    end_s5=end_s4*end_s;
    A=[1,start_s,start_s2,start_s3,start_s4,start_s5;
       0,1,2*start_s,3*start_s2,4*start_s3,5*start_s4;
       0,0,2,6*start_s,12*start_s2,20*start_s3;
       1,end_s,end_s2,end_s3,end_s4,end_s5;
       0,1,2*end_s,3*end_s2,4*end_s3,5*end_s4;
        0,0,2,6*end_s,12*end_s2,20*end_s3;];
    B=[start_l;start_dl;start_ddl;end_l;end_dl;end_ddl];
    coffee=A\B;
end

== matlab function testemplanner_cs/Audi_A8_Sedan_1/decision&planning module/EM_planner1/path decision with dynamic planning(dp) ==
  data: obs_s_set input; dp_path_s output; obs_l_set input; plan_start_s input; plan_start_l input; plan_start_dl input; plan_start_dll input; w_cost_collision input; w_cost_smooth_dl input; w_cost_smooth_ddl input; w_cost_smooth_dddl input; w_cost_ref input; row input; col input; sample_s input; sample_l input; dp_path_l output
function [dp_path_s,dp_path_l] = fcn(obs_s_set,obs_l_set,plan_start_s,plan_start_l,plan_start_dl,...
    plan_start_dll,w_cost_collision,w_cost_smooth_dl,w_cost_smooth_ddl,w_cost_smooth_dddl,w_cost_ref,row,col,sample_s,sample_l)
%该函数为路径决策算法动态规划的主函数
% 输入：obs s l set 筛选后的障碍物sl信息
%       plan_start s l dl ddl 规划起点信息
%       w_cost_obs,w_cost_smooth_dl,w_cost_smooth_ddl,w_cost_smooth_dddl,w_cost_ref动态规划代价权重
%       row col 动态规划采样点的行数和列数(row必须是奇数，col必须是6)
%       sample_s,sample_l 采样的s l 长度
% 输出：dp_path_l,dp_path_s 动态规划的路径sl,此路径不包含规划起点  

%动态规划最优的数据结构是结构体矩阵，但是simulink不支持结构体矩阵，所以动态规划算法写的相对难以理解

%声明二维矩阵变量node_cost，node_cost(i,j)表示从起点出发，到行i列j节点的最小代价为node_cost(i,j)
node_cost = ones(row,col)*inf;%初始化为无穷大

%声明二维矩阵变量pre_node_index pre_node_index(i,j)表示从起点到行i列j的节点的最优路径中前一个节点的行号为
%pre_node_index(i,j)
%例：比如一条最优路径为 起点 -> node(1,1) -> node(2,2) -> node(3,3)
%则pre_node_index(3,3) = 2 (最优路径的前一个节点是node(2,2) 取它的行号）
%  pre_node_index(2,2) = 1 (最优路径的前一个节点是node(1,1) 取它的行号）
%  pre_node_index(1,1) = 0 (起点的行号默认是0)

% 其实pre_node_index就是当找到最小代价的路径后从终点到起点反向选择出最优路径的
%如果用结构体矩阵完全没有必要弄得这么麻烦，但是simulink不支持
pre_node_index = zeros(row,col);%初始化，所有节点的上个最优节点的行号都是0，也就是起点

%先计算从起点到第一列的cost
for i = 1:row
    node_cost(i,1) = CalcStartCost(plan_start_s,plan_start_l,plan_start_dl,...
    plan_start_dll,i,sample_s,sample_l,w_cost_collision,w_cost_smooth_dl,...
    w_cost_smooth_ddl,w_cost_smooth_dddl,w_cost_ref,obs_s_set,obs_l_set,row);
end
% 动态规划主函数，从第二列开始
for j = 2:col
    for i = 1:row
        %计算当前node(i,j)的s l
        cur_node_s = plan_start_s + j * sample_s;
        cur_node_l = ((row + 1)/2 - i) * sample_l;
        %遍历前一列的节点
        for k = 1:row
            %计算前一列节点的s l
            pre_node_s = plan_start_s + (j - 1) * sample_s;
            pre_node_l = ((row + 1)/2 - k) * sample_l;
            cost_neighbour = CalcNeighbourCost(pre_node_s,pre_node_l,cur_node_s,cur_node_l,w_cost_collision,...
    w_cost_smooth_dl,w_cost_smooth_ddl,w_cost_smooth_dddl,w_cost_ref,obs_s_set,obs_l_set);
            %起点到上一个节点的最小代价为node_cost(k,j-1)
            pre_min_cost = node_cost(k,j-1);
            %起点到node_cost(i,j)的最小代价 为node_cost(k,j-1)
            %再加上node(k,j-1)到node(i,j)的代价 (k = 1,2,3,4...row) 中最小的
            cost_temp = pre_min_cost + cost_neighbour;
            if cost_temp < node_cost(i,j)
                node_cost(i,j) = cost_temp;
                %把最优路径上一列节点的行号记录下来
                pre_node_index(i,j) = k;
            end
        end      
    end
end
%找到node_cost最后一列中，cost最小的，记代价最小的行号为index
index = 0;
min_cost = inf;
for i = 1:row
    if node_cost(i,end) < min_cost
        min_cost = node_cost(i,end);
        index = i;
    end
end
%动态规划最优路径初始化
dp_node_list_row = zeros(col,1);
%从后往前逆推
cur_index = index;
for i = 1:col
    %记录cur_index前面节点的行号
    pre_index = pre_node_index(cur_index,end - i + 1);
    %把cur_index放到dp_node_list_row对应的位置
    dp_node_list_row(col - i + 1) = cur_index;
    %再把pre_index 赋给 cur_index 进行下一步递推
    cur_index = pre_index;
end
% 输出初始化，由于事先不知道横纵向的采样列数，因此需要做缓冲
dp_path_s = ones(15,1)*-1;
dp_path_l = ones(15,1)*-1;
for i = 1:col
    dp_path_s(i) = plan_start_s + i * sample_s;
    dp_path_l(i) = ((row + 1) / 2 - dp_node_list_row(i)) * sample_l;
end








end
function cost = CalcNeighbourCost(pre_node_s,pre_node_l,cur_node_s,cur_node_l,w_cost_collision,...
    w_cost_smooth_dl,w_cost_smooth_ddl,w_cost_smooth_dddl,w_cost_ref,obs_s_set,obs_l_set)
% 该函数将计算相邻两个节点之间的cost
  
    start_l = pre_node_l;
    start_dl = 0;
    start_ddl = 0;
    end_l = cur_node_l;
    end_dl = 0;
    end_ddl = 0;
    start_s = pre_node_s;
    end_s = cur_node_s;
    coeff = CalcQuinticCoeffient(start_l,start_dl,start_ddl,end_l,end_dl,end_ddl,start_s,end_s);
    a0 = coeff(1);
    a1 = coeff(2);
    a2 = coeff(3);
    a3 = coeff(4);
    a4 = coeff(5);
    a5 = coeff(6);
    % 取10个点计算cost
    ds = zeros(10,1);
    l = zeros(10,1);
    dl = zeros(10,1);
    ddl = zeros(10,1);
    dddl = zeros(10,1);
    for i = 1:10
        ds(i) = start_s + (i-1)*(end_s - start_s)/10;
    end
    l = a0 * ones(10,1) + a1 * ds + a2 * ds.^2 + a3 * ds.^3 + a4 * ds.^4 + a5 * ds.^5;
    dl = a1 * ones(10,1) + 2 * a2 * ds + 3 * a3 * ds.^2 + 4 * a4 * ds.^3 + 5 * a5 * ds.^4;
    ddl = 2 * a2 * ones(10,1) + 6 * a3 * ds + 12 * a4 * ds.^2 + 20 * a5 * ds.^3;
    dddl = 6 * ones(10,1) * a3 + 24 * a4 * ds + 60 * a5 * ds.^2;
    cost_smooth = w_cost_smooth_dl * (dl' * dl) + w_cost_smooth_ddl * (ddl' * ddl) + w_cost_smooth_dddl * (dddl' * dddl);
    cost_ref = w_cost_ref * (l' * l);
    cost_collision = 0;
    for i = 1:length(obs_s_set)
        if isnan(obs_s_set(i))
            break;
        end
        dlon = ones(10,1) * obs_s_set(i) - ds;
        dlat = ones(10,1) * obs_l_set(i) - l;
        %这里做了非常简化的质点模型，认为障碍物就是一个点
        square_d = dlon.^2 + dlat.^2;
        cost_collision_once = CalcObsCost(w_cost_collision,square_d);
        cost_collision = cost_collision + cost_collision_once;
    end
    cost = cost_collision + cost_smooth + cost_ref;


end


function cost = CalcStartCost(begin_s,begin_l,begin_dl,begin_ddl,cur_node_row,sample_s,sample_l,w_cost_collision,...
    w_cost_smooth_dl,w_cost_smooth_ddl,w_cost_smooth_dddl,w_cost_ref,obs_s_set,obs_l_set,row)
    %该函数将计算起点到第一层的cost
    start_l = begin_l;
    start_dl = begin_dl;
    start_ddl = begin_ddl;
    %  . . .
    %  . . . row = 3 中间的行号 = (row + 1) /2 = 2
    %  . . .
    end_l = ((row + 1)/2 - cur_node_row)*sample_l;
    end_dl = 0;
    end_ddl = 0;
    start_s = begin_s;
    end_s = begin_s + sample_s;
    coeff = CalcQuinticCoeffient(start_l,start_dl,start_ddl,end_l,end_dl,end_ddl,start_s,end_s);
    a0 = coeff(1);
    a1 = coeff(2);
    a2 = coeff(3);
    a3 = coeff(4);
    a4 = coeff(5);
    a5 = coeff(6);
    % 取10个点计算cost
    ds = zeros(10,1);
    l = zeros(10,1);
    dl = zeros(10,1);
    ddl = zeros(10,1);
    dddl = zeros(10,1);
    for i = 1:10
        ds(i) = start_s + (i-1)*sample_s/10;
    end
    l = a0 * ones(10,1) + a1 * ds + a2 * ds.^2 + a3 * ds.^3 + a4 * ds.^4 + a5 * ds.^5;
    dl = a1 * ones(10,1) + 2 * a2 * ds + 3 * a3 * ds.^2 + 4 * a4 * ds.^3 + 5 * a5 * ds.^4;
    ddl = 2 * a2 * ones(10,1) + 6 * a3 * ds + 12 * a4 * ds.^2 + 20 * a5 * ds.^3;
    dddl = 6 * ones(10,1) * a3 + 24 * a4 * ds + 60 * a5 * ds.^2;
    cost_smooth = w_cost_smooth_dl * (dl' * dl) + w_cost_smooth_ddl * (ddl' * ddl) + w_cost_smooth_dddl * (dddl' * dddl);
    cost_ref = w_cost_ref * (l' * l);
    cost_collision = 0;
    for i = 1:length(obs_s_set)
        if isnan(obs_s_set(i))
            break;
        end
        dlon = ones(10,1) * obs_s_set(i) - ds;
        dlat = ones(10,1) * obs_l_set(i) - l;
        %这里做了非常简化的质点模型，认为障碍物就是一个点
        square_d = dlon.^2 + dlat.^2;
        cost_collision_once = CalcObsCost(w_cost_collision,square_d);
        cost_collision = cost_collision + cost_collision_once;
    end
    cost = cost_collision + cost_smooth + cost_ref;
        
end

function obs_cost = CalcObsCost(w_cost_collision,square_d)
%该函数将计算障碍物的距离代价
% 暂定超过4米的cost为0 在4到3米的cost为1000/squard_d,在小于3米的cost为w_cost_collision
  cost = 0;
  for i = 1:length(square_d)
      if (square_d(i) < 16 && square_d(i) > 9) 
          cost = cost + 1000/square_d(i);
      elseif (square_d(i) < 9)
          cost = cost + w_cost_collision;
      end
  end
  obs_cost = cost;

end

function coeff = CalcQuinticCoeffient(start_l,start_dl,start_ddl,end_l,end_dl,end_ddl,start_s,end_s)
    % l = a0 + a1*s + a2*s^2 + a3*s^3 + a4*s^4 + a5*s^5
    % l' = a1 + 2 * a2 * s + 3 * a3 * s^2 + 4 * a4 * s^3 + 5 * a5 * s^4
    % l'' = 2 * a2 + 6 * a3 * s + 12 * a4 * s^2 + 20 * a5 * s^3
    start_s2 = start_s * start_s;
    start_s3 = start_s2 * start_s;
    start_s4 = start_s3 * start_s;
    start_s5 = start_s4 * start_s;
    end_s2 = end_s * end_s;
    end_s3 = end_s2 * end_s;
    end_s4 = end_s3 * end_s;
    end_s5 = end_s4 * end_s;
   
     A=[1,start_s,start_s2,start_s3,start_s4,start_s5;
       0,1,2*start_s,3*start_s2,4*start_s3,5*start_s4;
       0,0,2,6*start_s,12*start_s2,20*start_s3;
       1,end_s,end_s2,end_s3,end_s4,end_s5;
       0,1,2*end_s,3*end_s2,4*end_s3,5*end_s4;
        0,0,2,6*end_s,12*end_s2,20*end_s3;];
    B=[start_l;start_dl;start_ddl;end_l;end_dl;end_ddl];
     coeff = A \ B;
    
end
